simulink model "LQR_estimare"  (R2023b)
settings: Solver=VariableStepAuto  StartTime=0.0  StopTime=120  RelTol=1e-3
values from neighbouring files (symbols this model uses):
  A = [0 lambda 0 0 ... (first row only)    [rotary_inverted_pendulum.m]    (also in sis_liniar.m)
  B = [0; B21; 0; B41]./lambda    [rotary_inverted_pendulum.m]    (also in sis_liniar.m)
  C = [0 0 1 0]    [rotary_inverted_pendulum.m]
  K = lqr(A,B,Q,R)    [rotary_inverted_pendulum.m]
  N = -inv(C*inv(A-B*K)*B)    [rotary_inverted_pendulum.m]
settings Model: Creator=ovidiuceoca  LastModifiedBy=ovidiuceoca

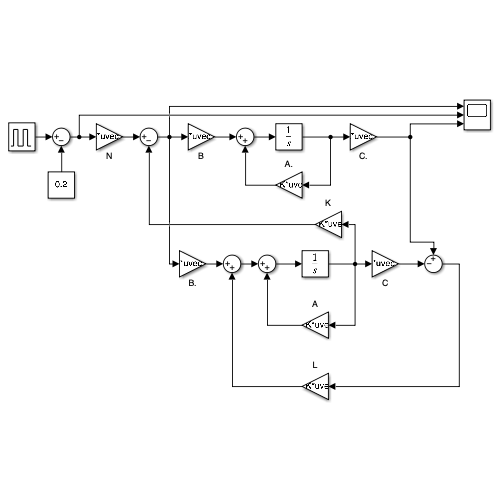
[thumbnail: Simulink's stored preview of the top-level diagram]
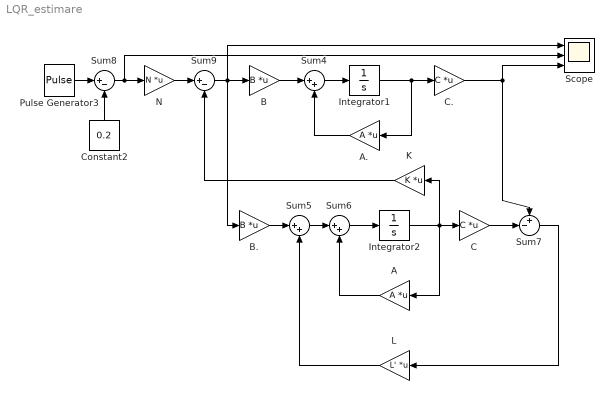
== system LQR_estimare ==
  A : Gain  Gain=A  Multiplication=Matrix(K*u) (u vector)
  A. : Gain  Gain=A  Multiplication=Matrix(K*u) (u vector)
  B : Gain  Gain=B  Multiplication=Matrix(K*u) (u vector)
  B. : Gain  Gain=B  Multiplication=Matrix(K*u) (u vector)
  C : Gain  Gain=C  Multiplication=Matrix(K*u) (u vector)
  C. : Gain  Gain=C  Multiplication=Matrix(K*u) (u vector)
  Constant2 : Constant  Value=0.2
  Integrator1 : Integrator
  Integrator2 : Integrator  InitialCondition=[1,1,1,1]
  K : Gain  Gain=K  Multiplication=Matrix(K*u) (u vector)
  L : Gain  Gain=L'  Multiplication=Matrix(K*u) (u vector)
  N : Gain  Gain=N  Multiplication=Matrix(K*u) (u vector)
  Pulse Generator3 : DiscretePulseGenerator  PulseType=Time based  Amplitude=1.5  Period=30  PulseWidth=50  PhaseDelay=15
  Scope : Scope  NumInputPorts=3
  Sum4 : Sum  Inputs=|++
  Sum5 : Sum  Inputs=|++
  Sum6 : Sum  Inputs=|++
  Sum7 : Sum  Inputs=+-|
  Sum8 : Sum  Inputs=|+-
  Sum9 : Sum  Inputs=|+-
  wires:
  Sum5/1 -> Sum6/1
  K/1 -> Sum9/2
  Sum4/1 -> Integrator1/1
  C./1 -> Scope/3, Sum7/1
  B/1 -> Sum4/1
  Sum7/1 -> L/1
  C/1 -> Sum7/2
  A./1 -> Sum4/2
  N/1 -> Sum9/1
  Pulse Generator3/1 -> Sum8/1
  Sum6/1 -> Integrator2/1
  A/1 -> Sum6/2
  L/1 -> Sum5/2
  Constant2/1 -> Sum8/2
  B./1 -> Sum5/1
  Sum8/1 -> Scope/2, N/1
  Sum9/1 -> Scope/1, B/1, B./1
  Integrator2/1 -> K/1, C/1, A/1
  Integrator1/1 -> A./1, C./1
